simulink model "ampc_cstr_estimation"  (R2022a)
settings: Solver=ode45  StartTime=0  StopTime=150  MaxStep=0.5*Ts  RelTol=1e-3  EnableMultiTasking=on
values from neighbouring files (symbols this model uses):
  Ts = 0.5    [ampccstr_estimation.m]
  u0 = [op_report.Inputs(1).u;op_report.Inputs(2).u;op_report.Inputs(3).u]    [ampccstr_estimation.m]
  x0 = [op_report.States(1).x;op_report.States(2).x]    [ampccstr_estimation.m]
  y0 = [op_report.Outputs(1).y;op_report.Outputs(2).y]    [ampccstr_estimation.m]
libraries: slident x2, mpclib x1, simulink x1
settings Model: Creator=The MathWorks, Inc.  LastModifiedBy=arkiven4
settings SolverCC: AlgebraicLoopSolver=TrustRegion
settings DataIOCC: ExternalInput=ExtIn  InitialState=[311.267; 8.5695]  SaveFormat=Structure  SaveOutput=off  SignalLogging=off  DSMLogging=off  SaveTime=off  ReturnWorkspaceOutputs=off  SignalLoggingName=logsOut
settings OptimizationCC: BooleanDataType=off  DefaultParameterBehavior=Inlined  InlineInvariantSignals=on  BufferReuse=off  ExpressionDepthLimit=2147483647  InitFltsAndDblsToZero=on  LifeSpan=inf
settings DebuggingCC: SaveWithParameterizedLinksMsg=none  UnderspecifiedInitializationDetection=Classic  MergeDetectMultiDrivingBlocksExec=none  CheckExecutionContextPreStartOutputMsg=on  SignalResolutionControl=TryResolveAllWithWarning  MultiTaskDSMMsg=warning  MultiTaskCondExecSysMsg=none  UnconnectedInputMsg=warning  UnconnectedOutputMsg=warning  UnconnectedLineMsg=warning  StateNameClashWarn=warning  SFUnexpectedBacktrackingDiag=warning  SFNoUnconditionalDefaultTransitionDiag=warning  SFExecutionAtInitializationDiag=none  SFMachineParentedDataDiag=warning  ArithmeticOperatorsInVariantConditions=warning
settings HardwareCC: ProdBitPerPointer=32  ProdBitPerSizeT=32  ProdBitPerPtrDiffT=32  ProdLargestAtomicFloat=None  ProdIntDivRoundTo=Undefined  ProdEndianess=Unspecified  ProdWordSize=32  ProdHWDeviceType=32-bit Generic  TargetUnknown=on
settings ModelReferenceCC: PropagateSignalLabelsOutOfModel=off
settings SFSimCC: SimUseLocalCustomCode=off  CustomCodeUndefinedFunction=UseInterfaceOnly
settings RTWCC: RTWUseLocalCustomCode=off
settings CodeAppCC: StateflowObjectComments=on
settings GRTTargetCC: TargetFcnLib=ansi_tfl_tmw.mat  TargetLangStandard=C89/C90 (ANSI)  CombineOutputUpdateFcns=off  GRTInterface=on
settings ConfigComp: CovMetricSettings=dw  CovSaveCumulativeToWorkspaceVar=on  CovSaveSingleToWorkspaceVar=on  CovExternalEMLEnable=off  CovSFcnEnable=off

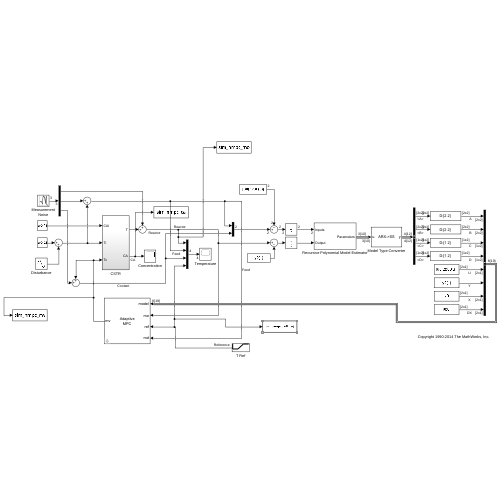
[thumbnail: Simulink's stored preview of the top-level diagram]
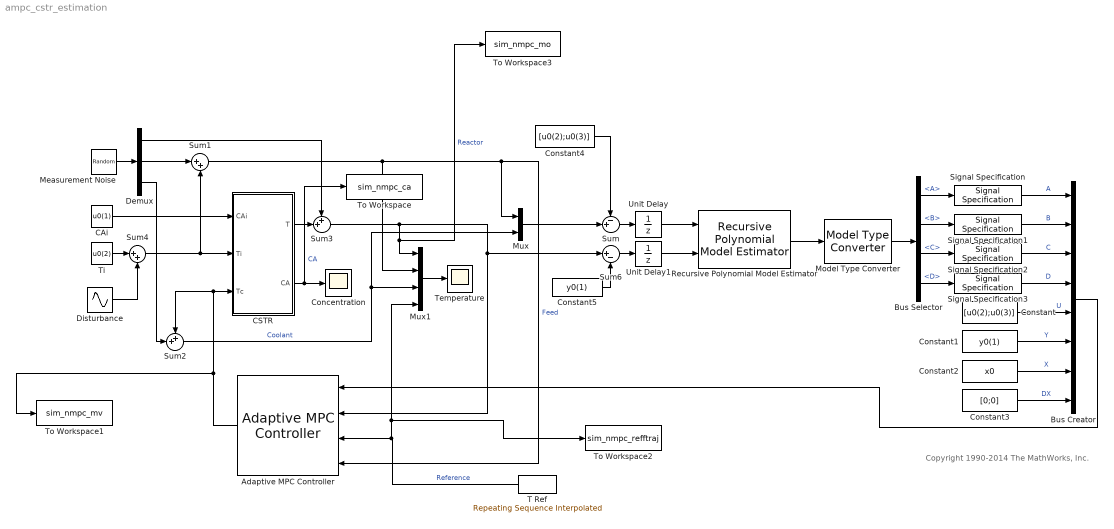
== system ampc_cstr_estimation ==
  note: Copyright 1990-2014 The MathWorks, Inc.
  Adaptive MPC Controller : mpclib/Adaptive MPC Controller  SCDEnableBlockLinearizationSpecification=on  mpcobj=mpcobj  enable_value=0  updateMPCinCallerWorkspace=on  md_inport=on  mv_inport=off  uref_inport=off  return_cost=off  return_mvseq=off  return_qpstatus=off  return_xseq=off  return_state=off  return_ovseq=off  state_inport=off  isltv_plant=off  umin_inport=off  umax_inport=off  ymin_inport=off  ymax_inport=off  cc_inport=off  ywt_inport=off  uwt_inport=off  duwt_inport=off  rhoeps_inport=off  pm_inport=off  MaximumP=10  HorizonChoice=FixedHorizon  BlockDataType=double  SampleTimeInherited=off  switch_inport=off
  Bus Creator : BusCreator  Inputs=8
  Bus Selector : BusSelector  OutputSignals=A,B,C,D
  CAi : Constant  Value=u0(1)
  CSTR : Subsystem
  Concentration : Scope
  Constant : Constant  Value=[u0(2);u0(3)]  VectorParams1D=off
  Constant1 : Constant  Value=y0(1)  VectorParams1D=off
  Constant2 : Constant  Value=x0  VectorParams1D=off
  Constant3 : Constant  Value=[0;0]  VectorParams1D=off
  Constant4 : Constant  Value=[u0(2);u0(3)]
  Constant5 : Constant  Value=y0(1)
  Demux : Demux  Outputs=3
  Disturbance : Sin  Amplitude=5  Frequency=0.05  SampleTime=0
  Measurement Noise : RandomNumber  Mean=[0 0 0]  Variance=0.001*[1 1 1]  Seed=12345  SampleTime=Ts/5
  Model Type Converter : slident/Estimators/Model Type Converter  InputModelType=ARX
      settings: SourceProductBaseCode=ID
  Mux : Mux  Inputs=2
  Mux1 : Mux
  Recursive Polynomial Model Estimator : slident/Estimators/Recursive Polynomial Model Estimator  ModelStructure=ARX  InitialEstimateSource=Internal  A0=Aq  B0=Bq  C0=1  D0=1  F0=1  nk=1  P0=1  InitialInputs=0  InitialOutputs=0  History=Infinite  WindowLength=200  EstimationMethod=Kalman Filter  AdaptationParameter=0.01  HasTimeVaryingAdaptationParameter=off  NormalizationBias=eps  OutputError=off  OutputP=off  AddEnablePort=off  InputProcessing=Sample-based  Ts=Ts
      settings: SourceProductBaseCode=ID
  Signal Specification : SignalSpecification  Dimensions=[2 2]
  Signal Specification1 : SignalSpecification  Dimensions=[2 2]
  Signal Specification2 : SignalSpecification  Dimensions=[1 2]
  Signal Specification3 : SignalSpecification  Dimensions=[1 2]
  Sum : Sum  Inputs=-+|
  Sum1 : Sum  Inputs=|++  SampleTime=Ts/5
  Sum2 : Sum  Inputs=++|  SampleTime=Ts/5
  Sum3 : Sum  Inputs=++|  SampleTime=Ts/5
  Sum4 : Sum  Inputs=|++  SampleTime=Ts/5
  Sum6 : Sum  Inputs=|+-
  T Ref : simulink/Sources/Repeating Sequence Interpolated  OutValues=[y0(1) y0(1) 373 373]  TimeValues=[0 50 100 150]  LookUpMeth=Interpolation-Use End Values  tsamp=Ts  OutMin=[]  OutMax=[]  OutDataTypeStr=double  OutputDataTypeScalingMode=double  OutDataType=fixdt(0,8)  OutScaling=2^-10
  Temperature : Scope
  Ti : Constant  Value=u0(2)
  To Workspace : ToWorkspace  VariableName=sim_nmpc_ca  SaveFormat=Timeseries  SampleTime=-1
  To Workspace1 : ToWorkspace  VariableName=sim_nmpc_mv  SaveFormat=Timeseries  SampleTime=-1
  To Workspace2 : ToWorkspace  VariableName=sim_nmpc_refftraj  SaveFormat=Timeseries  SampleTime=-1
  To Workspace3 : ToWorkspace  VariableName=sim_nmpc_mo  SaveFormat=Timeseries  SampleTime=-1
  Unit Delay : UnitDelay  InitialCondition=[0;0]  SampleTime=Ts  HasFrameUpgradeWarning=on
  Unit Delay1 : UnitDelay  SampleTime=Ts  HasFrameUpgradeWarning=on
  wires:
  Mux1/1 -> Temperature/1
  Sum1/1 -> Adaptive MPC Controller/4, Mux/1, Mux1/2  "Feed"
  Bus Creator/1 -> Adaptive MPC Controller/1
  Sum2/1 -> Mux/2, Mux1/3  "Coolant"
  Sum3/1 -> Adaptive MPC Controller/2, Sum6/1, To Workspace3/1, Mux1/1  "Reactor"
  CSTR/2(CA) -> To Workspace/1, Concentration/1  "CA"
  CSTR/1(T) -> Sum3/2
  Ti/1 -> Sum4/1
  Sum4/1 -> Sum1/2, CSTR/2(Ti)
  Disturbance/1 -> Sum4/2
  Demux/2 -> Sum1/1
  Demux/1 -> Sum3/1
  Demux/3 -> Sum2/2
  Measurement Noise/1 -> Demux/1
  Unit Delay1/1 -> Recursive Polynomial Model Estimator/2
  Model Type Converter/1 -> Bus Selector/1
  Recursive Polynomial Model Estimator/1 -> Model Type Converter/1
  Constant1/1 -> Bus Creator/6  "Y"
  Constant/1 -> Bus Creator/5  "U"
  Bus Selector/1 -> Signal Specification/1  "<A>"
  Signal Specification/1 -> Bus Creator/1  "A"
  Bus Selector/2 -> Signal Specification1/1  "<B>"
  Bus Selector/3 -> Signal Specification2/1  "<C>"
  Bus Selector/4 -> Signal Specification3/1  "<D>"
  Signal Specification1/1 -> Bus Creator/2  "B"
  Signal Specification2/1 -> Bus Creator/3  "C"
  Signal Specification3/1 -> Bus Creator/4  "D"
  Constant2/1 -> Bus Creator/7  "X"
  Constant3/1 -> Bus Creator/8  "DX"
  Sum6/1 -> Unit Delay1/1
  Sum/1 -> Unit Delay/1
  Mux/1 -> Sum/2
  Constant4/1 -> Sum/1
  Unit Delay/1 -> Recursive Polynomial Model Estimator/1
  Constant5/1 -> Sum6/2
  CAi/1 -> CSTR/1(CAi)
  Adaptive MPC Controller/1 -> To Workspace1/1, CSTR/3(Tc), Sum2/1
  T Ref/1 -> To Workspace2/1, Mux1/4, Adaptive MPC Controller/3  "Reference"

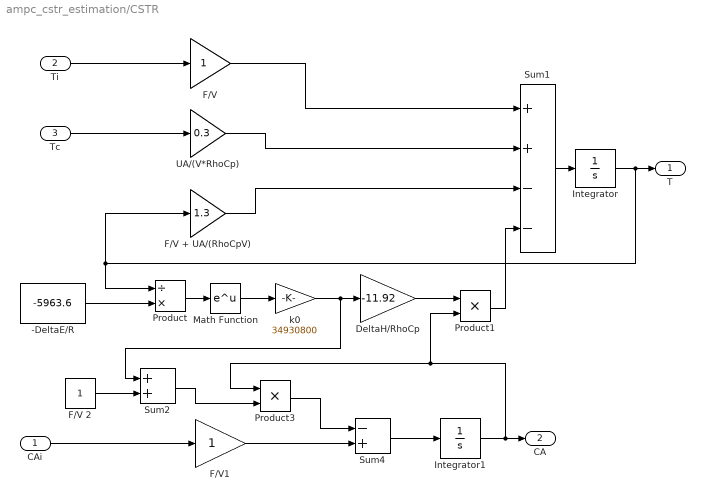
== system ampc_cstr_estimation/CSTR ==
  CAi : Inport
  Ti : Inport  Port=2
  Tc : Inport  Port=3
  -DeltaE/R : Constant  Value=-5963.6
  DeltaH/RhoCp : Gain  Gain=-11.92  SaturateOnIntegerOverflow=on  OutDataTypeStr=Inherit: Same as input  ParamDataTypeStr=Inherit: Same as input
  F/V : Gain  SaturateOnIntegerOverflow=on  OutDataTypeStr=Inherit: Same as input  ParamDataTypeStr=Inherit: Same as input
  F/V + UA/(RhoCpV) : Gain  Gain=1.3  SaturateOnIntegerOverflow=on  OutDataTypeStr=Inherit: Same as input  ParamDataTypeStr=Inherit: Same as input
  F/V 2 : Constant
  F/V1 : Gain  SaturateOnIntegerOverflow=on  OutDataTypeStr=Inherit: Same as input  ParamDataTypeStr=Inherit: Same as input
  Integrator : Integrator  InitialCondition=311.2639  LimitOutput=on  LowerSaturationLimit=0
  Integrator1 : Integrator  InitialCondition=8.5698  LimitOutput=on  LowerSaturationLimit=0
  Math Function : Math  SignedPower=on
  Product : Product  Inputs=/*  InputSameDT=on  RndMeth=Zero  SaturateOnIntegerOverflow=on  OutDataTypeStr=Inherit: Same as first input
  Product1 : Product  InputSameDT=on  RndMeth=Zero  SaturateOnIntegerOverflow=on  OutDataTypeStr=Inherit: Same as first input
  Product3 : Product  InputSameDT=on  RndMeth=Zero  SaturateOnIntegerOverflow=on  OutDataTypeStr=Inherit: Same as first input
  Sum1 : Sum  Inputs=++--  InputSameDT=on  SaturateOnIntegerOverflow=on  OutDataTypeStr=Inherit: Same as first input
  Sum2 : Sum  InputSameDT=on  SaturateOnIntegerOverflow=on  OutDataTypeStr=Inherit: Same as first input
  Sum4 : Sum  Inputs=-+  InputSameDT=on  SaturateOnIntegerOverflow=on  OutDataTypeStr=Inherit: Same as first input
  UA/(V*RhoCp) : Gain  Gain=0.3  SaturateOnIntegerOverflow=on  OutDataTypeStr=Inherit: Same as input  ParamDataTypeStr=Inherit: Same as input
  k0 : Gain  Gain=34930800  SaturateOnIntegerOverflow=on  OutDataTypeStr=Inherit: Same as input  ParamDataTypeStr=Inherit: Same as input
  T : Outport  VectorParamsAs1DForOutWhenUnconnected=off
  CA : Outport  Port=2  VectorParamsAs1DForOutWhenUnconnected=off
  wires:
  Sum2/1 -> Product3/2
  Tc/1 -> UA/(V*RhoCp)/1
  CAi/1 -> F/V1/1
  Ti/1 -> F/V/1
  F/V1/1 -> Sum4/2
  F/V 2/1 -> Sum2/2
  Integrator1/1 -> CA/1, Product3/1, Product1/2
  Sum4/1 -> Integrator1/1
  Product3/1 -> Sum4/1
  -DeltaE/R/1 -> Product/2
  k0/1 -> Sum2/1, DeltaH/RhoCp/1
  Product1/1 -> Sum1/4
  DeltaH/RhoCp/1 -> Product1/1
  Math Function/1 -> k0/1
  Product/1 -> Math Function/1
  F/V + UA/(RhoCpV)/1 -> Sum1/3
  UA/(V*RhoCp)/1 -> Sum1/2
  Integrator/1 -> T/1, F/V + UA/(RhoCpV)/1, Product/1
  Sum1/1 -> Integrator/1
  F/V/1 -> Sum1/1
